simulink model "SimLink03"  (R2021a)
settings: Solver=VariableStepAuto  StartTime=0.0  StopTime=10.0  RelTol=1e-3
libraries: commsrccod2 x2, dspsrcs4 x1
settings Model: Creator=lefs3303  LastModifiedBy=lefs3303

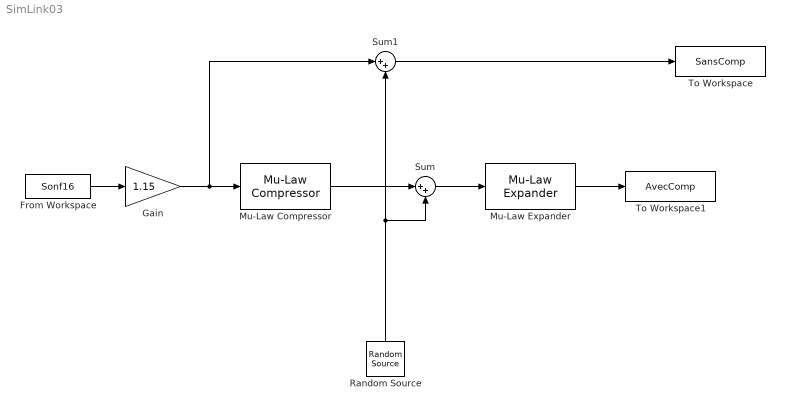
== system SimLink03 ==
  From Workspace : FromWorkspace  VariableName=Sonf16  SampleTime=1/16000
  Gain : Gain  Gain=1.15
  Mu-Law Compressor : commsrccod2/Mu-Law Compressor  mu=255  V=1
      settings: SourceProductBaseCode=CM
  Mu-Law Expander : commsrccod2/Mu-Law Expander  mu=255  V=1
      settings: SourceProductBaseCode=CM
  Random Source : dspsrcs4/Random Source  SrcType=Gaussian  NormMethod=Ziggurat  CltLength=12  MinVal=0  MaxVal=1  MeanVal=0  VarVal=0.048  RepMode=Not repeatable  rawSeed=1  IsInherit=off  SampMode=Discrete  SampTime=1/16000  SampFrame=1  DataType=Double  OutComplex=Real  OutputFrames=off
  Sum : Sum  Inputs=|++
  Sum1 : Sum  Inputs=|++
  To Workspace : ToWorkspace  VariableName=SansComp  SampleTime=-1
      settings: Save2DSignal=2-D array (concatenate along first dimension)
  To Workspace1 : ToWorkspace  VariableName=AvecComp  SampleTime=-1
      settings: Save2DSignal=2-D array (concatenate along first dimension)
  wires:
  From Workspace/1 -> Gain/1
  Gain/1 -> Sum1/1, Mu-Law Compressor/1
  Random Source/1 -> Sum/2, Sum1/2
  Sum1/1 -> To Workspace/1
  Mu-Law Compressor/1 -> Sum/1
  Sum/1 -> Mu-Law Expander/1
  Mu-Law Expander/1 -> To Workspace1/1
